simulink model "Assembly_union"  (R2020a)
settings: Solver=VariableStepAuto  StartTime=0.0  StopTime=inf  RelTol=1e-3
model workspace: external: MATLAB File A:\Usuarios\TATTO PC\Desktop\univesidad\Procesamiento video y audio\proyecto 6 intelingencia artificial\Assembly3_DataFile.m (data not in the file)
undefined symbols (not defined in the file or in its folder): smiData, X, Y, Z
libraries: neural x563, sm_lib x153, nesl_utility x4, dspstat3 x3, audiosources x1, simulink x1, dspxfrm3 x1
(part 3 of 36)

== system Assembly_union/Assembly_zona_1/l31_1_RIGID ==
  ReferenceFrame : sm_lib/Frames and Transforms/Reference Frame
  Solid : sm_lib/Body Elements/File Solid  ExtGeomFileName=l31.step  UnitType=FromFile  ExtGeomFileUnits=m  StepReaderType=HEX  ExportConvexHullGeometry=off  InertiaType=Custom  Mass=1  MassUnits=kg  CenterOfMass=smiData.Solid(36).CoM  CenterOfMassUnits=mm  MomentsOfInertia=smiData.Solid(36).MoI  MomentsOfInertiaUnits=kg*mm^2  ProductsOfInertia=smiData.Solid(36).PoI  ProductsOfInertiaUnits=kg*mm^2  BasedOnType=DensityFromFile  Density=1000  DensityUnits=kg/m^3  DoExposeReferenceFrame=on  SerializedFrames=<Frames/>  GraphicType=FromGeometry  MarkerShape=Sphere  MarkerSize=10  GraphicVisPropType=SimpleVisualProperties  GraphicDiffuseColor=[1.0 0.8 0.0]  GraphicSpecularColor=[0.5 0.5 0.5 1.0]  GraphicAmbientColor=[0.15 0.15 0.15 1.0]  GraphicEmissiveColor=[0.0 0.0 0.0 1.0]  GraphicShininess=75  GraphicOpacity=smiData.Solid(36).opacity
  F : PMIOPort  Side=Left
  connections:
  Solid/RConn1 -- ReferenceFrame/RConn1 -- F/RConn1

== system Assembly_union/Assembly_zona_1/l32_1_RIGID ==
  ReferenceFrame : sm_lib/Frames and Transforms/Reference Frame
  Solid : sm_lib/Body Elements/File Solid  ExtGeomFileName=l32.step  UnitType=FromFile  ExtGeomFileUnits=m  StepReaderType=HEX  ExportConvexHullGeometry=off  InertiaType=Custom  Mass=1  MassUnits=kg  CenterOfMass=smiData.Solid(50).CoM  CenterOfMassUnits=mm  MomentsOfInertia=smiData.Solid(50).MoI  MomentsOfInertiaUnits=kg*mm^2  ProductsOfInertia=smiData.Solid(50).PoI  ProductsOfInertiaUnits=kg*mm^2  BasedOnType=DensityFromFile  Density=1000  DensityUnits=kg/m^3  DoExposeReferenceFrame=on  SerializedFrames=<Frames/>  GraphicType=FromGeometry  MarkerShape=Sphere  MarkerSize=10  GraphicVisPropType=SimpleVisualProperties  GraphicDiffuseColor=[1.0 0.8 0.0]  GraphicSpecularColor=[0.5 0.5 0.5 1.0]  GraphicAmbientColor=[0.15 0.15 0.15 1.0]  GraphicEmissiveColor=[0.0 0.0 0.0 1.0]  GraphicShininess=75  GraphicOpacity=smiData.Solid(50).opacity
  F : PMIOPort  Side=Left
  connections:
  Solid/RConn1 -- ReferenceFrame/RConn1 -- F/RConn1

== system Assembly_union/Assembly_zona_1/l41_1_RIGID ==
  ReferenceFrame : sm_lib/Frames and Transforms/Reference Frame
  Solid : sm_lib/Body Elements/File Solid  ExtGeomFileName=l41.step  UnitType=FromFile  ExtGeomFileUnits=m  StepReaderType=HEX  ExportConvexHullGeometry=off  InertiaType=Custom  Mass=1  MassUnits=kg  CenterOfMass=smiData.Solid(39).CoM  CenterOfMassUnits=mm  MomentsOfInertia=smiData.Solid(39).MoI  MomentsOfInertiaUnits=kg*mm^2  ProductsOfInertia=smiData.Solid(39).PoI  ProductsOfInertiaUnits=kg*mm^2  BasedOnType=DensityFromFile  Density=1000  DensityUnits=kg/m^3  DoExposeReferenceFrame=on  SerializedFrames=<Frames/>  GraphicType=FromGeometry  MarkerShape=Sphere  MarkerSize=10  GraphicVisPropType=SimpleVisualProperties  GraphicDiffuseColor=[1.0 0.8 0.0]  GraphicSpecularColor=[0.5 0.5 0.5 1.0]  GraphicAmbientColor=[0.15 0.15 0.15 1.0]  GraphicEmissiveColor=[0.0 0.0 0.0 1.0]  GraphicShininess=75  GraphicOpacity=smiData.Solid(39).opacity
  F : PMIOPort  Side=Left
  connections:
  Solid/RConn1 -- ReferenceFrame/RConn1 -- F/RConn1

== system Assembly_union/Assembly_zona_1/l42_1_RIGID ==
  ReferenceFrame : sm_lib/Frames and Transforms/Reference Frame
  Solid : sm_lib/Body Elements/File Solid  ExtGeomFileName=l42.step  UnitType=FromFile  ExtGeomFileUnits=m  StepReaderType=HEX  ExportConvexHullGeometry=off  InertiaType=Custom  Mass=1  MassUnits=kg  CenterOfMass=smiData.Solid(41).CoM  CenterOfMassUnits=mm  MomentsOfInertia=smiData.Solid(41).MoI  MomentsOfInertiaUnits=kg*mm^2  ProductsOfInertia=smiData.Solid(41).PoI  ProductsOfInertiaUnits=kg*mm^2  BasedOnType=DensityFromFile  Density=1000  DensityUnits=kg/m^3  DoExposeReferenceFrame=on  SerializedFrames=<Frames/>  GraphicType=FromGeometry  MarkerShape=Sphere  MarkerSize=10  GraphicVisPropType=SimpleVisualProperties  GraphicDiffuseColor=[1.0 0.8 0.0]  GraphicSpecularColor=[0.5 0.5 0.5 1.0]  GraphicAmbientColor=[0.15 0.15 0.15 1.0]  GraphicEmissiveColor=[0.0 0.0 0.0 1.0]  GraphicShininess=75  GraphicOpacity=smiData.Solid(41).opacity
  F : PMIOPort  Side=Left
  connections:
  Solid/RConn1 -- ReferenceFrame/RConn1 -- F/RConn1

== system Assembly_union/Assembly_zona_1/lineacentro_1_RIGID ==
  ReferenceFrame : sm_lib/Frames and Transforms/Reference Frame
  Solid : sm_lib/Body Elements/File Solid  ExtGeomFileName=lineacentro.step  UnitType=FromFile  ExtGeomFileUnits=m  StepReaderType=HEX  ExportConvexHullGeometry=off  InertiaType=Custom  Mass=1  MassUnits=kg  CenterOfMass=smiData.Solid(45).CoM  CenterOfMassUnits=mm  MomentsOfInertia=smiData.Solid(45).MoI  MomentsOfInertiaUnits=kg*mm^2  ProductsOfInertia=smiData.Solid(45).PoI  ProductsOfInertiaUnits=kg*mm^2  BasedOnType=DensityFromFile  Density=1000  DensityUnits=kg/m^3  DoExposeReferenceFrame=on  SerializedFrames=<Frames/>  GraphicType=FromGeometry  MarkerShape=Sphere  MarkerSize=10  GraphicVisPropType=SimpleVisualProperties  GraphicDiffuseColor=[1.0 0.8 0.0]  GraphicSpecularColor=[0.5 0.5 0.5 1.0]  GraphicAmbientColor=[0.15 0.15 0.15 1.0]  GraphicEmissiveColor=[0.0 0.0 0.0 1.0]  GraphicShininess=75  GraphicOpacity=smiData.Solid(45).opacity
  F : PMIOPort  Side=Left
  connections:
  Solid/RConn1 -- ReferenceFrame/RConn1 -- F/RConn1

== system Assembly_union/Assembly_zona_1/pasto1_1_RIGID ==
  ReferenceFrame : sm_lib/Frames and Transforms/Reference Frame
  Solid : sm_lib/Body Elements/File Solid  ExtGeomFileName=pasto1.step  UnitType=FromFile  ExtGeomFileUnits=m  StepReaderType=HEX  ExportConvexHullGeometry=off  InertiaType=Custom  Mass=1  MassUnits=kg  CenterOfMass=smiData.Solid(40).CoM  CenterOfMassUnits=mm  MomentsOfInertia=smiData.Solid(40).MoI  MomentsOfInertiaUnits=kg*mm^2  ProductsOfInertia=smiData.Solid(40).PoI  ProductsOfInertiaUnits=kg*mm^2  BasedOnType=DensityFromFile  Density=1000  DensityUnits=kg/m^3  DoExposeReferenceFrame=on  SerializedFrames=<Frames/>  GraphicType=FromGeometry  MarkerShape=Sphere  MarkerSize=10  GraphicVisPropType=SimpleVisualProperties  GraphicDiffuseColor=[0.2 0.6 0.0]  GraphicSpecularColor=[0.5 0.5 0.5 1.0]  GraphicAmbientColor=[0.15 0.15 0.15 1.0]  GraphicEmissiveColor=[0.0 0.0 0.0 1.0]  GraphicShininess=75  GraphicOpacity=smiData.Solid(40).opacity
  F : PMIOPort  Side=Left
  connections:
  Solid/RConn1 -- ReferenceFrame/RConn1 -- F/RConn1

== system Assembly_union/Assembly_zona_1/pasto2_1_RIGID ==
  ReferenceFrame : sm_lib/Frames and Transforms/Reference Frame
  Solid : sm_lib/Body Elements/File Solid  ExtGeomFileName=pasto2.step  UnitType=FromFile  ExtGeomFileUnits=m  StepReaderType=HEX  ExportConvexHullGeometry=off  InertiaType=Custom  Mass=1  MassUnits=kg  CenterOfMass=smiData.Solid(42).CoM  CenterOfMassUnits=mm  MomentsOfInertia=smiData.Solid(42).MoI  MomentsOfInertiaUnits=kg*mm^2  ProductsOfInertia=smiData.Solid(42).PoI  ProductsOfInertiaUnits=kg*mm^2  BasedOnType=DensityFromFile  Density=1000  DensityUnits=kg/m^3  DoExposeReferenceFrame=on  SerializedFrames=<Frames/>  GraphicType=FromGeometry  MarkerShape=Sphere  MarkerSize=10  GraphicVisPropType=SimpleVisualProperties  GraphicDiffuseColor=[0.2 0.6 0.0]  GraphicSpecularColor=[0.5 0.5 0.5 1.0]  GraphicAmbientColor=[0.15 0.15 0.15 1.0]  GraphicEmissiveColor=[0.0 0.0 0.0 1.0]  GraphicShininess=75  GraphicOpacity=smiData.Solid(42).opacity
  F : PMIOPort  Side=Left
  connections:
  Solid/RConn1 -- ReferenceFrame/RConn1 -- F/RConn1

== system Assembly_union/Assembly_zona_1/pasto4_1_RIGID ==
  ReferenceFrame : sm_lib/Frames and Transforms/Reference Frame
  Solid : sm_lib/Body Elements/File Solid  ExtGeomFileName=pasto4.step  UnitType=FromFile  ExtGeomFileUnits=m  StepReaderType=HEX  ExportConvexHullGeometry=off  InertiaType=Custom  Mass=1  MassUnits=kg  CenterOfMass=smiData.Solid(52).CoM  CenterOfMassUnits=mm  MomentsOfInertia=smiData.Solid(52).MoI  MomentsOfInertiaUnits=kg*mm^2  ProductsOfInertia=smiData.Solid(52).PoI  ProductsOfInertiaUnits=kg*mm^2  BasedOnType=DensityFromFile  Density=1000  DensityUnits=kg/m^3  DoExposeReferenceFrame=on  SerializedFrames=<Frames/>  GraphicType=FromGeometry  MarkerShape=Sphere  MarkerSize=10  GraphicVisPropType=SimpleVisualProperties  GraphicDiffuseColor=[0.2 0.6 0.0]  GraphicSpecularColor=[0.5 0.5 0.5 1.0]  GraphicAmbientColor=[0.15 0.15 0.15 1.0]  GraphicEmissiveColor=[0.0 0.0 0.0 1.0]  GraphicShininess=75  GraphicOpacity=smiData.Solid(52).opacity
  F : PMIOPort  Side=Left
  connections:
  Solid/RConn1 -- ReferenceFrame/RConn1 -- F/RConn1

== system Assembly_union/Assembly_zona_1/pasto5_1_RIGID ==
  ReferenceFrame : sm_lib/Frames and Transforms/Reference Frame
  Solid : sm_lib/Body Elements/File Solid  ExtGeomFileName=pasto5.step  UnitType=FromFile  ExtGeomFileUnits=m  StepReaderType=HEX  ExportConvexHullGeometry=off  InertiaType=Custom  Mass=1  MassUnits=kg  CenterOfMass=smiData.Solid(51).CoM  CenterOfMassUnits=mm  MomentsOfInertia=smiData.Solid(51).MoI  MomentsOfInertiaUnits=kg*mm^2  ProductsOfInertia=smiData.Solid(51).PoI  ProductsOfInertiaUnits=kg*mm^2  BasedOnType=DensityFromFile  Density=1000  DensityUnits=kg/m^3  DoExposeReferenceFrame=on  SerializedFrames=<Frames/>  GraphicType=FromGeometry  MarkerShape=Sphere  MarkerSize=10  GraphicVisPropType=SimpleVisualProperties  GraphicDiffuseColor=[0.2 0.6 0.0]  GraphicSpecularColor=[0.5 0.5 0.5 1.0]  GraphicAmbientColor=[0.15 0.15 0.15 1.0]  GraphicEmissiveColor=[0.0 0.0 0.0 1.0]  GraphicShininess=75  GraphicOpacity=smiData.Solid(51).opacity
  F : PMIOPort  Side=Left
  connections:
  Solid/RConn1 -- ReferenceFrame/RConn1 -- F/RConn1

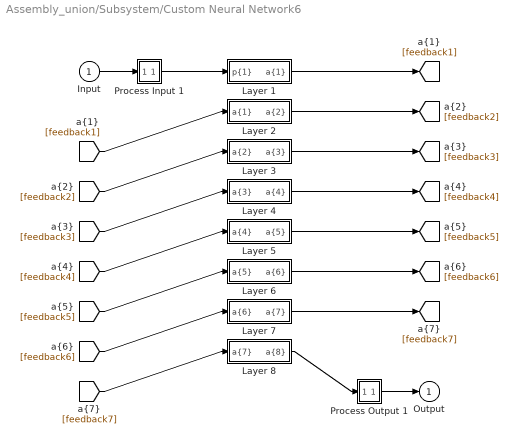
== system Assembly_union/Subsystem/Custom Neural Network6 ==
  Input : Inport  PortDimensions=63
      mask Display: e = 0.06;c1 = [120 230 180]/255;c2 = ([120 230 180]+0)/(256+128);c3 = ([120 230 180]+128)/(256+128);patch([0 1 1 0],[0 0 1 1],c1);patch([0 1 1 1-e 1-e 0+e],[0 0 1 1-e 0+e 0+e],c2);patch([0 0 1 1-e 0+e 0+e],[0 1 1 1-e 1-e 0+e],c3);plot([0 1 1 0 0],[0 0 1 1 0]);
  Layer 1 : Subsystem
      mask Display: e = 0.06;c1 = [120 150 230]/255;c2 = ([120 150 230]+0)/383;c3 = ([120 150 230]+128)/383;patch([0 1 1 0],[0 0 1 1],c1);patch([0 1 1 1-e 1-e 0+e],[0 0 1 1-e 0+e 0+e],c2);patch([0 0 1 1-e 0+e 0+e],[0 1 1 1-e 1-e 0+e],c3);plot([0 1 1 0 0],[0 0 1 1 0]);
  Layer 2 : Subsystem
      mask Display: e = 0.06;c1 = [120 150 230]/255;c2 = ([120 150 230]+0)/383;c3 = ([120 150 230]+128)/383;patch([0 1 1 0],[0 0 1 1],c1);patch([0 1 1 1-e 1-e 0+e],[0 0 1 1-e 0+e 0+e],c2);patch([0 0 1 1-e 0+e 0+e],[0 1 1 1-e 1-e 0+e],c3);plot([0 1 1 0 0],[0 0 1 1 0]);
  Layer 3 : Subsystem
      mask Display: e = 0.06;c1 = [120 150 230]/255;c2 = ([120 150 230]+0)/383;c3 = ([120 150 230]+128)/383;patch([0 1 1 0],[0 0 1 1],c1);patch([0 1 1 1-e 1-e 0+e],[0 0 1 1-e 0+e 0+e],c2);patch([0 0 1 1-e 0+e 0+e],[0 1 1 1-e 1-e 0+e],c3);plot([0 1 1 0 0],[0 0 1 1 0]);
  Layer 4 : Subsystem
      mask Display: e = 0.06;c1 = [120 150 230]/255;c2 = ([120 150 230]+0)/383;c3 = ([120 150 230]+128)/383;patch([0 1 1 0],[0 0 1 1],c1);patch([0 1 1 1-e 1-e 0+e],[0 0 1 1-e 0+e 0+e],c2);patch([0 0 1 1-e 0+e 0+e],[0 1 1 1-e 1-e 0+e],c3);plot([0 1 1 0 0],[0 0 1 1 0]);
  Layer 5 : Subsystem
      mask Display: e = 0.06;c1 = [120 150 230]/255;c2 = ([120 150 230]+0)/383;c3 = ([120 150 230]+128)/383;patch([0 1 1 0],[0 0 1 1],c1);patch([0 1 1 1-e 1-e 0+e],[0 0 1 1-e 0+e 0+e],c2);patch([0 0 1 1-e 0+e 0+e],[0 1 1 1-e 1-e 0+e],c3);plot([0 1 1 0 0],[0 0 1 1 0]);
  Layer 6 : Subsystem
      mask Display: e = 0.06;c1 = [120 150 230]/255;c2 = ([120 150 230]+0)/383;c3 = ([120 150 230]+128)/383;patch([0 1 1 0],[0 0 1 1],c1);patch([0 1 1 1-e 1-e 0+e],[0 0 1 1-e 0+e 0+e],c2);patch([0 0 1 1-e 0+e 0+e],[0 1 1 1-e 1-e 0+e],c3);plot([0 1 1 0 0],[0 0 1 1 0]);
  Layer 7 : Subsystem
      mask Display: e = 0.06;c1 = [120 150 230]/255;c2 = ([120 150 230]+0)/383;c3 = ([120 150 230]+128)/383;patch([0 1 1 0],[0 0 1 1],c1);patch([0 1 1 1-e 1-e 0+e],[0 0 1 1-e 0+e 0+e],c2);patch([0 0 1 1-e 0+e 0+e],[0 1 1 1-e 1-e 0+e],c3);plot([0 1 1 0 0],[0 0 1 1 0]);
  Layer 8 : Subsystem
      mask Display: e = 0.06;c1 = [120 150 230]/255;c2 = ([120 150 230]+0)/383;c3 = ([120 150 230]+128)/383;patch([0 1 1 0],[0 0 1 1],c1);patch([0 1 1 1-e 1-e 0+e],[0 0 1 1-e 0+e 0+e],c2);patch([0 0 1 1-e 0+e 0+e],[0 1 1 1-e 1-e 0+e],c3);plot([0 1 1 0 0],[0 0 1 1 0]);
  Process Input 1 : Subsystem
      mask Display: e = 0.06;c1 = [120 150 230]/255;c2 = ([120 150 230]+0)/383;c3 = ([120 150 230]+128)/383;patch([0 1 1 0],[0 0 1 1],c1);patch([0 1 1 1-e 1-e 0+e],[0 0 1 1-e 0+e 0+e],c2);patch([0 0 1 1-e 0+e 0+e],[0 1 1 1-e 1-e 0+e],c3);plot([0 1 1 0 0],[0 0 1 1 0]);
  Process Output 1 : Subsystem
      mask Display: e = 0.06;c1 = [120 150 230]/255;c2 = ([120 150 230]+0)/383;c3 = ([120 150 230]+128)/383;patch([0 1 1 0],[0 0 1 1],c1);patch([0 1 1 1-e 1-e 0+e],[0 0 1 1-e 0+e 0+e],c2);patch([0 0 1 1-e 0+e 0+e],[0 1 1 1-e 1-e 0+e],c3);plot([0 1 1 0 0],[0 0 1 1 0]);
  Output : Outport  InitialOutput=[0;0;0;0;0;0;0;0;0;0;0;0;0;0;0;0;0;0;0;0;0;0;0;0;0;0;0;0;0;0;0;0;0;0;0;0;0;0;0;0;0;0;0;0;0;0;0;0;0;0;0;0;0;0;0;0;0;0;0;0;0;0;0]
      mask Display: e = 0.06;c1 = [120 230 180]/255;c2 = ([120 230 180]+0)/(256+128);c3 = ([120 230 180]+128)/(256+128);patch([0 1 1 0],[0 0 1 1],c1);patch([0 1 1 1-e 1-e 0+e],[0 0 1 1-e 0+e 0+e],c2);patch([0 0 1 1-e 0+e 0+e],[0 1 1 1-e 1-e 0+e],c3);plot([0 1 1 0 0],[0 0 1 1 0]);
  wires:
  Input/1 -> Process Input 1/1(x)
  Process Output 1/1(y) -> Output/1
  Process Input 1/1(p) -> Layer 1/1("p{1}")
  Layer 1/1("a{1}") -> [feedback1]
  [feedback1] -> Layer 2/1("a{1} ")
  Layer 2/1("a{2}") -> [feedback2]
  [feedback2] -> Layer 3/1("a{2} ")
  Layer 3/1("a{3}") -> [feedback3]
  [feedback3] -> Layer 4/1("a{3} ")
  Layer 4/1("a{4}") -> [feedback4]
  [feedback4] -> Layer 5/1("a{4} ")
  Layer 5/1("a{5}") -> [feedback5]
  [feedback5] -> Layer 6/1("a{5} ")
  Layer 6/1("a{6}") -> [feedback6]
  [feedback6] -> Layer 7/1("a{6} ")
  Layer 7/1("a{7}") -> [feedback7]
  [feedback7] -> Layer 8/1("a{7} ")
  Layer 8/1("a{8}") -> Process Output 1/1(a)

== system Assembly_union/Subsystem/Custom Neural Network6/Layer 1 ==
  "p{1}" : Inport  PortDimensions=63
      mask Display: e = 0.06;c1 = [120 230 180]/255;c2 = ([120 230 180]+0)/(256+128);c3 = ([120 230 180]+128)/(256+128);patch([0 1 1 0],[0 0 1 1],c1);patch([0 1 1 1-e 1-e 0+e],[0 0 1 1-e 0+e 0+e],c2);patch([0 0 1 1-e 0+e 0+e],[0 1 1 1-e 1-e 0+e],c3);plot([0 1 1 0 0],[0 0 1 1 0]);
  Delays 1 : Subsystem
      mask Display: e = 0.06;c1 = [120 150 230]/255;c2 = ([120 150 230]+0)/383;c3 = ([120 150 230]+128)/383;patch([0 1 1 0],[0 0 1 1],c1);patch([0 1 1 1-e 1-e 0+e],[0 0 1 1-e 0+e 0+e],c2);patch([0 0 1 1-e 0+e 0+e],[0 1 1 1-e 1-e 0+e],c3);plot([0 1 1 0 0],[0 0 1 1 0]);disp('0');
  "IW{1,1}" : Subsystem
      mask Display: e = 0.06;c1 = [120 150 230]/255;c2 = ([120 150 230]+0)/383;c3 = ([120 150 230]+128)/383;patch([0 1 1 0],[0 0 1 1],c1);patch([0 1 1 1-e 1-e 0+e],[0 0 1 1-e 0+e 0+e],c2);patch([0 0 1 1-e 0+e 0+e],[0 1 1 1-e 1-e 0+e],c3);plot([0 1 1 0 0],[0 0 1 1 0]);disp('W');
  "b{1}" : Constant  Value=[-1.550357727038423671928057956392876803874969482421875;1.4470399743728241670481793335056863725185394287109375;-1.4617342382418410107192130453768186271190643310546875;1.3544264579599758491212924127466976642608642578125;-1.332780594198820001139438318205066025257110595703125;-1.281869263495257538210125858313404023647308349609375;-1.2429855642347249489176874703844077885150909423828125;1.1965614301382865303224889430566690862178802490234375;1.150447237016904100670444677234627306461334228515625;1.1076856284415625975015018411795608699321746826171875;-1.0671947287690344285948640390415675938129425048828125;-1.0218377385453776273749326719553209841251373291015625;0.9791302377141992696607530888286419212818145751953125;-0.92970916794972235930316628582659177482128143310546875;0.88277326608969708399143883070792071521282196044921875;0.85259394630971219175563646786031313240528106689453125;-0.797070887827824758886663403245620429515838623046875;0.7627876456740059207817239439464174211025238037109375;0.7170558634775912043579637611401267349720001220703125;0.68509918117150625516131867698277346789836883544921875;-0.657791786147828627662192957359366118907928466796875;0.5674359665739194813482981771812774240970611572265625;-0.54259375737416493112874604776152409613132476806640625;-0.51667223145751706159245486560394056141376495361328125;-0.454104607036566798594634519758983515202999114990234375;-0.41485030802403743965811599991866387426853179931640625;-0.35684593574554834827239346850547008216381072998046875;0.32771899110818070166573079404770396649837493896484375;0.25727155434146009582718761521391570568084716796875;-0.2334452069519412920062251259878394193947315216064453125;-0.1877030549718397001157654813141562044620513916015625;0.15072051773341854641330428421497344970703125;-0.10889311824829679686832406559915398247539997100830078125;0.050491628255018468351966731688662548549473285675048828125;0.0192865747800914366649749354110099375247955322265625;-0.022123242606346064931255313013025443069636821746826171875;-0.05263233856318709491528551325245643965899944305419921875;-0.11632565292821432645364865265946718864142894744873046875;0.1708024797534551109112754829766345210373401641845703125;0.1878478259147150775110191034400486387312412261962890625;-0.2442854221391420888043199965977692045271396636962890625;-0.2809311906560338911731378175318241119384765625;-0.322760707928959167389848516904748976230621337890625;-0.369668965987821118712730594779714010655879974365234375;-0.41898239754938793044658496000920422375202178955078125;0.458632299767689488589894608594477176666259765625;0.495758476221943078510179248041822575032711029052734375;-0.51115983647028973013703989636269398033618927001953125;-0.5699831976077576189965157027472741901874542236328125;0.6242764405988110443246341674239374697208404541015625;0.69164310496723213628200710445526055991649627685546875;-0.705583374553743869483923845109529793262481689453125;-0.77264797713766519837719215502147562801837921142578125;-0.793747601233798061315383165492676198482513427734375;0.82215014987183610006837852779426611959934234619140625;0.88353905011437616767722147415042854845523834228515625;-0.9455945735740918234313312495942227542400360107421875;-0.99019652083277076570766439544968307018280029296875;1.0171662055149415238020083052106201648712158203125;1.0700968569369597727103382567293010652065277099609375;-1.1381989868155120149140202556736767292022705078125;-1.15638637640822761198933221749030053615570068359375;-1.2248723353568939931079739835695363581180572509765625;1.2403596519018755817143073727493174374103546142578125;1.2795648758247690768286020102095790207386016845703125;1.321774707896936629225592696457169950008392333984375;-1.3745608698744093967292201341479085385799407958984375;1.4229278619727352417356769365142099559307098388671875;-1.4703002760689154460038707838975824415683746337890625;1.530732570996612640357170675997622311115264892578125]
      mask Display: e = 0.06;c1 = [120 150 230]/255;c2 = ([120 150 230]+0)/383;c3 = ([120 150 230]+128)/383;patch([0 1 1 0],[0 0 1 1],c1);patch([0 1 1 1-e 1-e 0+e],[0 0 1 1-e 0+e 0+e],c2);patch([0 0 1 1-e 0+e 0+e],[0 1 1 1-e 1-e 0+e],c3);plot([0 1 1 0 0],[0 0 1 1 0]);disp('b');
  netsum : Sum  Inputs=2  InputSameDT=on  SaturateOnIntegerOverflow=on  OutDataTypeStr=Inherit: Same as first input
      mask Display: e = 0.06;c1 = [120 150 230]/255;c2 = ([120 150 230]+0)/383;c3 = ([120 150 230]+128)/383;patch([0 1 1 0],[0 0 1 1],c1);patch([0 1 1 1-e 1-e 0+e],[0 0 1 1-e 0+e 0+e],c2);patch([0 0 1 1-e 0+e 0+e],[0 1 1 1-e 1-e 0+e],c3);plot([0 1 1 0 0],[0 0 1 1 0]);disp('+');
  tansig : neural/Transfer Functions/tansig
  "a{1}" : Outport  InitialOutput=[0;0;0;0;0;0;0;0;0;0;0;0;0;0;0;0;0;0;0;0;0;0;0;0;0;0;0;0;0;0;0;0;0;0;0;0;0;0;0;0;0;0;0;0;0;0;0;0;0;0;0;0;0;0;0;0;0;0;0;0;0;0;0;0;0;0;0;0;0;0]
      mask Display: e = 0.06;c1 = [120 230 180]/255;c2 = ([120 230 180]+0)/(256+128);c3 = ([120 230 180]+128)/(256+128);patch([0 1 1 0],[0 0 1 1],c1);patch([0 1 1 1-e 1-e 0+e],[0 0 1 1-e 0+e 0+e],c2);patch([0 0 1 1-e 0+e 0+e],[0 1 1 1-e 1-e 0+e],c3);plot([0 1 1 0 0],[0 0 1 1 0]);
  wires:
  "p{1}"/1 -> Delays 1/1("p{1}")
  Delays 1/1("pd{1,1}") -> "IW{1,1}"/1("pd{1,1}")
  "IW{1,1}"/1("iz{1,1}") -> netsum/1
  "b{1}"/1 -> netsum/2
  netsum/1 -> tansig/1
  tansig/1 -> "a{1}"/1

== system Assembly_union/Subsystem/Custom Neural Network6/Layer 2 ==
  "a{1} " : Inport  PortDimensions=70
      mask Display: e = 0.06;c1 = [120 230 180]/255;c2 = ([120 230 180]+0)/(256+128);c3 = ([120 230 180]+128)/(256+128);patch([0 1 1 0],[0 0 1 1],c1);patch([0 1 1 1-e 1-e 0+e],[0 0 1 1-e 0+e 0+e],c2);patch([0 0 1 1-e 0+e 0+e],[0 1 1 1-e 1-e 0+e],c3);plot([0 1 1 0 0],[0 0 1 1 0]);
  Delays 1 : Subsystem
      mask Display: e = 0.06;c1 = [120 150 230]/255;c2 = ([120 150 230]+0)/383;c3 = ([120 150 230]+128)/383;patch([0 1 1 0],[0 0 1 1],c1);patch([0 1 1 1-e 1-e 0+e],[0 0 1 1-e 0+e 0+e],c2);patch([0 0 1 1-e 0+e 0+e],[0 1 1 1-e 1-e 0+e],c3);plot([0 1 1 0 0],[0 0 1 1 0]);disp('0');
  "LW{2,1}" : Subsystem
      mask Display: e = 0.06;c1 = [120 150 230]/255;c2 = ([120 150 230]+0)/383;c3 = ([120 150 230]+128)/383;patch([0 1 1 0],[0 0 1 1],c1);patch([0 1 1 1-e 1-e 0+e],[0 0 1 1-e 0+e 0+e],c2);patch([0 0 1 1-e 0+e 0+e],[0 1 1 1-e 1-e 0+e],c3);plot([0 1 1 0 0],[0 0 1 1 0]);disp('W');
  "b{2}" : Constant  Value=[1.486726141153912994496977262315340340137481689453125;-1.4442907853435773546380005427636206150054931640625;-1.3994382199420620782603918996755965054035186767578125;1.3639489940170228532423379874671809375286102294921875;-1.313064173078837715280542397522367537021636962890625;-1.253979722265409879611297583323903381824493408203125;1.2320309107327209741100659812218509614467620849609375;-1.1994843709907707651751707089715637266635894775390625;1.1415421256358466717273358881357125937938690185546875;-1.1132711162864368237279677487094886600971221923828125;-1.0368331200875104958214478756417520344257354736328125;1.0218351117924004967107975971885025501251220703125;-0.94548852289680607174915394352865405380725860595703125;-0.939163356491530265657274867407977581024169921875;-0.89687245952084293509898316187900491058826446533203125;-0.84208100302565169759105856428504921495914459228515625;-0.79008406747387860402653814162476919591426849365234375;0.7504057562187711472034834514488466084003448486328125;0.69951147721582784821947598175029270350933074951171875;0.66872624632760935270425761700607836246490478515625;0.61790533552333026801051119036856107413768768310546875;-0.5964692178183546023007011172012425959110260009765625;-0.55270373980923126477904361308901570737361907958984375;-0.494761620773593591149364101511309854686260223388671875;-0.459687958993470979773832141290768049657344818115234375;-0.382591923718393400744020027559599839150905609130859375;0.374736436947102402594822478931746445596218109130859375;0.32834752417064116958300701298867352306842803955078125;-0.259761298706372822930887878101202659308910369873046875;0.243978329773085478304750495226471684873104095458984375;-0.2013183391247168885218599143627216108143329620361328125;-0.135075152550246435634306862993980757892131805419921875;0.09967379369076879991329320773729705251753330230712890625;0.07715536331574927852994250088158878497779369354248046875;0.0254663908700082895764094104151809005998075008392333984375;0.01311071261576543349469670118878639186732470989227294921875;0.08649478978454593069979949859771295450627803802490234375;-0.10679916289935420525836207161773927509784698486328125;0.1416173543784224053698750367402681149542331695556640625;-0.1978407897073064802828668007350643165409564971923828125;0.23368078724311602822893974007456563413143157958984375;0.28895186307564257877089630710543133318424224853515625;-0.325627842263375433251582080629304982721805572509765625;-0.356037176580408232240415600244887173175811767578125;0.423914235533638883435259003817918710410594940185546875;0.449368997809631298689936329537886194884777069091796875;0.50535496942426993971508863978669978678226470947265625;0.55113055039301439563814710709266364574432373046875;0.59100823243280931063026173433172516524791717529296875;-0.6352041961439887085560940249706618487834930419921875;0.66847616649831997914787962145055644214153289794921875;-0.7075611568129236417235006229020655155181884765625;-0.7386605460025419400693635907373391091823577880859375;0.80406440989228122884213689758325926959514617919921875;0.83301432776110073685771340024075470864772796630859375;0.85832211339386343951218805159442126750946044921875;0.9101257219447835833392446147627197206020355224609375;-0.93686181191686301872323383577167987823486328125;-1.01666218669575147970363104832358658313751220703125;-1.057844876234991904340176915866322815418243408203125;-1.1089896128049208101629119482822716236114501953125;1.1414191925987697828759337426163256168365478515625;-1.1843126675446791207235719411983154714107513427734375;1.2263680992950691805987162297242321074008941650390625;1.2703890144356531077818317498895339667797088623046875;-1.3185457817037036232221680620568804442882537841796875;1.3587844545992304734483013817225582897663116455078125;1.4039510047143723969753636993118561804294586181640625;-1.44427349025922868719362668343819677829742431640625;1.472144176816463367885035040671937167644500732421875]
      mask Display: e = 0.06;c1 = [120 150 230]/255;c2 = ([120 150 230]+0)/383;c3 = ([120 150 230]+128)/383;patch([0 1 1 0],[0 0 1 1],c1);patch([0 1 1 1-e 1-e 0+e],[0 0 1 1-e 0+e 0+e],c2);patch([0 0 1 1-e 0+e 0+e],[0 1 1 1-e 1-e 0+e],c3);plot([0 1 1 0 0],[0 0 1 1 0]);disp('b');
  netsum : Sum  Inputs=2  InputSameDT=on  SaturateOnIntegerOverflow=on  OutDataTypeStr=Inherit: Same as first input
      mask Display: e = 0.06;c1 = [120 150 230]/255;c2 = ([120 150 230]+0)/383;c3 = ([120 150 230]+128)/383;patch([0 1 1 0],[0 0 1 1],c1);patch([0 1 1 1-e 1-e 0+e],[0 0 1 1-e 0+e 0+e],c2);patch([0 0 1 1-e 0+e 0+e],[0 1 1 1-e 1-e 0+e],c3);plot([0 1 1 0 0],[0 0 1 1 0]);disp('+');
  tansig : neural/Transfer Functions/tansig
  "a{2}" : Outport  InitialOutput=[0;0;0;0;0;0;0;0;0;0;0;0;0;0;0;0;0;0;0;0;0;0;0;0;0;0;0;0;0;0;0;0;0;0;0;0;0;0;0;0;0;0;0;0;0;0;0;0;0;0;0;0;0;0;0;0;0;0;0;0;0;0;0;0;0;0;0;0;0;0]
      mask Display: e = 0.06;c1 = [120 230 180]/255;c2 = ([120 230 180]+0)/(256+128);c3 = ([120 230 180]+128)/(256+128);patch([0 1 1 0],[0 0 1 1],c1);patch([0 1 1 1-e 1-e 0+e],[0 0 1 1-e 0+e 0+e],c2);patch([0 0 1 1-e 0+e 0+e],[0 1 1 1-e 1-e 0+e],c3);plot([0 1 1 0 0],[0 0 1 1 0]);
  wires:
  "a{1} "/1 -> Delays 1/1("p{2}")
  Delays 1/1("pd{2,1}") -> "LW{2,1}"/1("ad{2,1}")
  "LW{2,1}"/1("lz{2,1}") -> netsum/1
  "b{2}"/1 -> netsum/2
  netsum/1 -> tansig/1
  tansig/1 -> "a{2}"/1

== system Assembly_union/Subsystem/Custom Neural Network6/Layer 3 ==
  "a{2} " : Inport  PortDimensions=70
      mask Display: e = 0.06;c1 = [120 230 180]/255;c2 = ([120 230 180]+0)/(256+128);c3 = ([120 230 180]+128)/(256+128);patch([0 1 1 0],[0 0 1 1],c1);patch([0 1 1 1-e 1-e 0+e],[0 0 1 1-e 0+e 0+e],c2);patch([0 0 1 1-e 0+e 0+e],[0 1 1 1-e 1-e 0+e],c3);plot([0 1 1 0 0],[0 0 1 1 0]);
  Delays 1 : Subsystem
      mask Display: e = 0.06;c1 = [120 150 230]/255;c2 = ([120 150 230]+0)/383;c3 = ([120 150 230]+128)/383;patch([0 1 1 0],[0 0 1 1],c1);patch([0 1 1 1-e 1-e 0+e],[0 0 1 1-e 0+e 0+e],c2);patch([0 0 1 1-e 0+e 0+e],[0 1 1 1-e 1-e 0+e],c3);plot([0 1 1 0 0],[0 0 1 1 0]);disp('0');
  "LW{3,2}" : Subsystem
      mask Display: e = 0.06;c1 = [120 150 230]/255;c2 = ([120 150 230]+0)/383;c3 = ([120 150 230]+128)/383;patch([0 1 1 0],[0 0 1 1],c1);patch([0 1 1 1-e 1-e 0+e],[0 0 1 1-e 0+e 0+e],c2);patch([0 0 1 1-e 0+e 0+e],[0 1 1 1-e 1-e 0+e],c3);plot([0 1 1 0 0],[0 0 1 1 0]);disp('W');
  "b{3}" : Constant  Value=[-1.478712157836084895023986973683349788188934326171875;-1.44204025517263811906332193757407367229461669921875;-1.406160436295465832046147625078447163105010986328125;1.349848375515560139348281154525466263294219970703125;1.3156653068339687617793742901994846761226654052734375;-1.2762747774459175520433973360923118889331817626953125;-1.216296923068817203983371655340306460857391357421875;-1.1936907194513113328326880946406163275241851806640625;1.1221280139287930222025124749052338302135467529296875;-1.0837860130475418518614105778397060930728912353515625;1.0362053873025127703755288166576065123081207275390625;-1.0085725426768890056195004945038817822933197021484375;0.97819503990188894082535853158333338797092437744140625;0.92446207740053953916259388279286213219165802001953125;-0.8904274695234712933000764678581617772579193115234375;-0.84085790275626559608923571431660093367099761962890625;0.78919718103128222441711159262922592461109161376953125;-0.75497647689017532979249835989321582019329071044921875;-0.70744719782572296207234785470063798129558563232421875;-0.67212498236491058367647610793937928974628448486328125;0.62391315929321589095479794195853173732757568359375;-0.58838687733364880561026666327961720526218414306640625;0.557943690780818624119774540304206311702728271484375;0.484293768076833830438232553206034936010837554931640625;-0.466714954829699102401008303786511532962322235107421875;0.408588143869419162523826116739655844867229461669921875;-0.370041780411621779034447854428435675799846649169921875;0.317845037801988639092343191805412061512470245361328125;0.285718702158025250614770129686803556978702545166015625;0.2279027705901833511514809060827246867120265960693359375;0.197681625942910443871625147949089296162128448486328125;0.141639221770150924850639739815960638225078582763671875;0.10991122798684893613341273521655239164829254150390625;-0.08405459902338958955159142760749091394245624542236328125;0.0254161748108656902755964068774119368754327297210693359375;0.0030851085640731580085616148068083930411376059055328369140625;-0.053561414881620007799600813314100378192961215972900390625;-0.1067284117360653705741668773043784312903881072998046875;-0.1420466952227823487220348397386260330677032470703125;-0.178821125963351257315281372939352877438068389892578125;-0.245904734168106264835529373158351518213748931884765625;0.27256549324913847964779733956675045192241668701171875;0.346085716802969900474096220932551659643650054931640625;0.36829035823397660021072397285024635493755340576171875;0.42602159858964927519053844662266783416271209716796875;-0.4433163274960831845561415320844389498233795166015625;-0.487373773709561197708950430751428939402103424072265625;-0.52597012896472083998133939530816860496997833251953125;0.5918245858972175366119472528225742280483245849609375;0.611382544474934785938557979534380137920379638671875;-0.6259379549411037135797641894896514713764190673828125;0.725374415083548829130677404464222490787506103515625;0.75450668920123253879950198097503744065761566162109375;0.79674844577210013341073135961778461933135986328125;-0.84047164760560078011764062466681934893131256103515625;0.88702752590263889143074038656777702271938323974609375;0.92346307374260250266928551354794763028621673583984375;-0.9718546289492600021020507483626715838909149169921875;1.0084743920896108715368200137163512408733367919921875;1.0673275480286650296335437815287150442600250244140625;-1.0968119710053993998144505894742906093597412109375;-1.142154966693210038641836945316754281520843505859375;1.188220600153555128741800217540003359317779541015625;-1.238418755972392926167913174140267074108123779296875;-1.2811983092021359542656000485294498503208160400390625;1.2971547567381327414892666638479568064212799072265625;-1.359799860984459929369450037484057247638702392578125;-1.40312044074937869453378880280070006847381591796875;1.4401144135696120063272473998949863016605377197265625;1.501471035054013913878634411958046257495880126953125]
      mask Display: e = 0.06;c1 = [120 150 230]/255;c2 = ([120 150 230]+0)/383;c3 = ([120 150 230]+128)/383;patch([0 1 1 0],[0 0 1 1],c1);patch([0 1 1 1-e 1-e 0+e],[0 0 1 1-e 0+e 0+e],c2);patch([0 0 1 1-e 0+e 0+e],[0 1 1 1-e 1-e 0+e],c3);plot([0 1 1 0 0],[0 0 1 1 0]);disp('b');
  netsum : Sum  Inputs=2  InputSameDT=on  SaturateOnIntegerOverflow=on  OutDataTypeStr=Inherit: Same as first input
      mask Display: e = 0.06;c1 = [120 150 230]/255;c2 = ([120 150 230]+0)/383;c3 = ([120 150 230]+128)/383;patch([0 1 1 0],[0 0 1 1],c1);patch([0 1 1 1-e 1-e 0+e],[0 0 1 1-e 0+e 0+e],c2);patch([0 0 1 1-e 0+e 0+e],[0 1 1 1-e 1-e 0+e],c3);plot([0 1 1 0 0],[0 0 1 1 0]);disp('+');
  tansig : neural/Transfer Functions/tansig
  "a{3}" : Outport  InitialOutput=[0;0;0;0;0;0;0;0;0;0;0;0;0;0;0;0;0;0;0;0;0;0;0;0;0;0;0;0;0;0;0;0;0;0;0;0;0;0;0;0;0;0;0;0;0;0;0;0;0;0;0;0;0;0;0;0;0;0;0;0;0;0;0;0;0;0;0;0;0;0]
      mask Display: e = 0.06;c1 = [120 230 180]/255;c2 = ([120 230 180]+0)/(256+128);c3 = ([120 230 180]+128)/(256+128);patch([0 1 1 0],[0 0 1 1],c1);patch([0 1 1 1-e 1-e 0+e],[0 0 1 1-e 0+e 0+e],c2);patch([0 0 1 1-e 0+e 0+e],[0 1 1 1-e 1-e 0+e],c3);plot([0 1 1 0 0],[0 0 1 1 0]);
  wires:
  "a{2} "/1 -> Delays 1/1("p{3}")
  Delays 1/1("pd{3,2}") -> "LW{3,2}"/1("ad{3,2}")
  "LW{3,2}"/1("lz{3,2}") -> netsum/1
  "b{3}"/1 -> netsum/2
  netsum/1 -> tansig/1
  tansig/1 -> "a{3}"/1

== system Assembly_union/Subsystem/Custom Neural Network6/Layer 4 ==
  "a{3} " : Inport  PortDimensions=70
      mask Display: e = 0.06;c1 = [120 230 180]/255;c2 = ([120 230 180]+0)/(256+128);c3 = ([120 230 180]+128)/(256+128);patch([0 1 1 0],[0 0 1 1],c1);patch([0 1 1 1-e 1-e 0+e],[0 0 1 1-e 0+e 0+e],c2);patch([0 0 1 1-e 0+e 0+e],[0 1 1 1-e 1-e 0+e],c3);plot([0 1 1 0 0],[0 0 1 1 0]);
  Delays 1 : Subsystem
      mask Display: e = 0.06;c1 = [120 150 230]/255;c2 = ([120 150 230]+0)/383;c3 = ([120 150 230]+128)/383;patch([0 1 1 0],[0 0 1 1],c1);patch([0 1 1 1-e 1-e 0+e],[0 0 1 1-e 0+e 0+e],c2);patch([0 0 1 1-e 0+e 0+e],[0 1 1 1-e 1-e 0+e],c3);plot([0 1 1 0 0],[0 0 1 1 0]);disp('0');
  "LW{4,3}" : Subsystem
      mask Display: e = 0.06;c1 = [120 150 230]/255;c2 = ([120 150 230]+0)/383;c3 = ([120 150 230]+128)/383;patch([0 1 1 0],[0 0 1 1],c1);patch([0 1 1 1-e 1-e 0+e],[0 0 1 1-e 0+e 0+e],c2);patch([0 0 1 1-e 0+e 0+e],[0 1 1 1-e 1-e 0+e],c3);plot([0 1 1 0 0],[0 0 1 1 0]);disp('W');
  "b{4}" : Constant  Value=[1.5076205391287189616633668265421874821186065673828125;-1.4454400764673935864124132422148250043392181396484375;-1.397161785664160493780627803062088787555694580078125;-1.3583220349444637964353432835196144878864288330078125;-1.3171629955426222835512817255221307277679443359375;-1.2654189831773283714255740051157772541046142578125;-1.225895245279738698940263930126093327999114990234375;-1.16834039096092556775374760036356747150421142578125;1.1468101635519019065867496465216390788555145263671875;1.09745774049859701193554428755305707454681396484375;1.0439516658008993754691573485615663230419158935546875;1.0185865979571440131934423334314487874507904052734375;-0.95641176497005264689477144202101044356822967529296875;0.91126947294328719539890926171210594475269317626953125;-0.886998331904802927994069250416941940784454345703125;-0.8234638924262582815316591222654096782207489013671875;-0.783363172959019582464179620728828012943267822265625;0.7483182450542980035379514447413384914398193359375;0.71774674395461068865387233017827384173870086669921875;0.66519349088265877778525236863060854375362396240234375;-0.62450948057194699547522986904368735849857330322265625;-0.56763313346006760706785598813439719378948211669921875;0.5194820002575102346753510573762468993663787841796875;-0.47033850536826482535701643428183160722255706787109375;-0.465320416039982698297450269819819368422031402587890625;-0.40050450986524654961584701595711521804332733154296875;0.366276252772025745496620174890267662703990936279296875;0.332853642976636165951020984721253626048564910888671875;0.29616859492819280763598044359241612255573272705078125;-0.244780544104318986686763537363731302320957183837890625;0.196628780808129732804445666261017322540283203125;-0.160227637155226310117228649687604047358036041259765625;-0.09925608451466851056554929755293414928019046783447265625;0.061610634172378477002585128730061114765703678131103515625;-0.0244463143815594301233584673127552377991378307342529296875;0.02553180005264481244875440779651398770511150360107421875;-0.0609366549343008656602904693500022403895854949951171875;0.11219979101187678438567019156835158355534076690673828125;0.1428638606575833580603074324244516901671886444091796875;0.1876276339611566701393030598410405218601226806640625;-0.252625530374786466669689843911328352987766265869140625;0.2767030950303703829007417880347929894924163818359375;0.339408720682780218336205280138528905808925628662109375;0.371622626067612926714645027459482662379741668701171875;-0.416631015628964818109380985333700664341449737548828125;0.456339399459154415605866006444557569921016693115234375;-0.478570635137376576562218133403803221881389617919921875;-0.539857403775162225656458758749067783355712890625;-0.58933904148836846470516093177138827741146087646484375;0.62058785035510666272529078923980705440044403076171875;-0.66293083572840505457435256175813265144824981689453125;0.7031424374129058296745142797590233385562896728515625;0.75467569143736057402094274948467500507831573486328125;-0.80091318161830304944714953307993710041046142578125;-0.8425541670021250428845860369619913399219512939453125;0.896203394914901974033227816107682883739471435546875;-0.93518123141223241656661002707551233470439910888671875;-0.97110822667775431593639723359956406056880950927734375;0.999815924799395627786680051940493285655975341796875;-1.057337551632094641007597601856105029582977294921875;-1.084754176438625261624792983639054000377655029296875;-1.1475994906122106709034369487199001014232635498046875;-1.1857505015850293705881313144345767796039581298828125;1.242192319077707995944592767045833170413970947265625;1.28533576171691610312564080231823027133941650390625;-1.315637352118816494339625933207571506500244140625;1.3621094318186919291946423982153646647930145263671875;-1.39768257197458733998018942656926810741424560546875;-1.44414663216938077283657548832707107067108154296875;-1.4781683970480152812143614937667734920978546142578125]
      mask Display: e = 0.06;c1 = [120 150 230]/255;c2 = ([120 150 230]+0)/383;c3 = ([120 150 230]+128)/383;patch([0 1 1 0],[0 0 1 1],c1);patch([0 1 1 1-e 1-e 0+e],[0 0 1 1-e 0+e 0+e],c2);patch([0 0 1 1-e 0+e 0+e],[0 1 1 1-e 1-e 0+e],c3);plot([0 1 1 0 0],[0 0 1 1 0]);disp('b');
  netsum : Sum  Inputs=2  InputSameDT=on  SaturateOnIntegerOverflow=on  OutDataTypeStr=Inherit: Same as first input
      mask Display: e = 0.06;c1 = [120 150 230]/255;c2 = ([120 150 230]+0)/383;c3 = ([120 150 230]+128)/383;patch([0 1 1 0],[0 0 1 1],c1);patch([0 1 1 1-e 1-e 0+e],[0 0 1 1-e 0+e 0+e],c2);patch([0 0 1 1-e 0+e 0+e],[0 1 1 1-e 1-e 0+e],c3);plot([0 1 1 0 0],[0 0 1 1 0]);disp('+');
  tansig : neural/Transfer Functions/tansig
  "a{4}" : Outport  InitialOutput=[0;0;0;0;0;0;0;0;0;0;0;0;0;0;0;0;0;0;0;0;0;0;0;0;0;0;0;0;0;0;0;0;0;0;0;0;0;0;0;0;0;0;0;0;0;0;0;0;0;0;0;0;0;0;0;0;0;0;0;0;0;0;0;0;0;0;0;0;0;0]
      mask Display: e = 0.06;c1 = [120 230 180]/255;c2 = ([120 230 180]+0)/(256+128);c3 = ([120 230 180]+128)/(256+128);patch([0 1 1 0],[0 0 1 1],c1);patch([0 1 1 1-e 1-e 0+e],[0 0 1 1-e 0+e 0+e],c2);patch([0 0 1 1-e 0+e 0+e],[0 1 1 1-e 1-e 0+e],c3);plot([0 1 1 0 0],[0 0 1 1 0]);
  wires:
  "a{3} "/1 -> Delays 1/1("p{4}")
  Delays 1/1("pd{4,3}") -> "LW{4,3}"/1("ad{4,3}")
  "LW{4,3}"/1("lz{4,3}") -> netsum/1
  "b{4}"/1 -> netsum/2
  netsum/1 -> tansig/1
  tansig/1 -> "a{4}"/1

== system Assembly_union/Subsystem/Custom Neural Network6/Layer 5 ==
  "a{4} " : Inport  PortDimensions=70
      mask Display: e = 0.06;c1 = [120 230 180]/255;c2 = ([120 230 180]+0)/(256+128);c3 = ([120 230 180]+128)/(256+128);patch([0 1 1 0],[0 0 1 1],c1);patch([0 1 1 1-e 1-e 0+e],[0 0 1 1-e 0+e 0+e],c2);patch([0 0 1 1-e 0+e 0+e],[0 1 1 1-e 1-e 0+e],c3);plot([0 1 1 0 0],[0 0 1 1 0]);
  Delays 1 : Subsystem
      mask Display: e = 0.06;c1 = [120 150 230]/255;c2 = ([120 150 230]+0)/383;c3 = ([120 150 230]+128)/383;patch([0 1 1 0],[0 0 1 1],c1);patch([0 1 1 1-e 1-e 0+e],[0 0 1 1-e 0+e 0+e],c2);patch([0 0 1 1-e 0+e 0+e],[0 1 1 1-e 1-e 0+e],c3);plot([0 1 1 0 0],[0 0 1 1 0]);disp('0');
  "LW{5,4}" : Subsystem
      mask Display: e = 0.06;c1 = [120 150 230]/255;c2 = ([120 150 230]+0)/383;c3 = ([120 150 230]+128)/383;patch([0 1 1 0],[0 0 1 1],c1);patch([0 1 1 1-e 1-e 0+e],[0 0 1 1-e 0+e 0+e],c2);patch([0 0 1 1-e 0+e 0+e],[0 1 1 1-e 1-e 0+e],c3);plot([0 1 1 0 0],[0 0 1 1 0]);disp('W');
  "b{5}" : Constant  Value=[1.4913534708448501486799386839265935122966766357421875;-1.4422974195684796772098934525274671614170074462890625;1.4017552719206129996365461920504458248615264892578125;-1.3457837262271115097433948903926648199558258056640625;-1.3178190209418598755064522265456616878509521484375;1.2677171267943923016474627729621715843677520751953125;1.2073010126882717241159070908906869590282440185546875;-1.1752189556032159867271502662333659827709197998046875;1.1450562194434088514327640950796194374561309814453125;1.1112574248288555889274675791966728866100311279296875;-1.057244907623533070051280446932651102542877197265625;1.046866471741549897700451765558682382106781005859375;-0.970099432584443643889926534029655158519744873046875;0.9233235668642552074203422307618893682956695556640625;-0.88387662237986341917661547995521686971187591552734375;-0.8566071450385168706276317607262171804904937744140625;-0.8012393797821377727785829847562126815319061279296875;-0.757196921632417030423312098719179630279541015625;0.71379591916863904810242047460633330047130584716796875;-0.692684139755799233029165407060645520687103271484375;0.6288687242091508533547994375112466514110565185546875;0.572504236613397221589139007846824824810028076171875;0.550432727718561221053050758200697600841522216796875;0.487460734204362144961208969107246957719326019287109375;-0.4361689822178098641103360932902432978153228759765625;0.417935347458838146739168450949364341795444488525390625;0.373930282203827790699079969272133894264698028564453125;-0.3160875626168007102023693732917308807373046875;-0.271998639184047930061893794118077494204044342041015625;-0.240315501627343497403899164055474102497100830078125;-0.2114422678490905649351105921596172265708446502685546875;-0.1494494749627695295846052658816915936768054962158203125;0.10931624238168570484308617096758098341524600982666015625;0.0629929819834859905380852751477505080401897430419921875;0.0254937841438631802859493546975500066764652729034423828125;-0.0428762284540773197516472237111884169280529022216796875;-0.0547400683400570964298736953423940576612949371337890625;0.10980104994544069574313738257842487655580043792724609375;-0.1629681992929138678594114253428415395319461822509765625;0.18650263243445486249783016319270245730876922607421875;-0.233303221912639024981928059787605889141559600830078125;-0.248728517698107609579238896913011558353900909423828125;-0.326036171763393556322085942156263627111911773681640625;0.347698569176673633052132572629489004611968994140625;-0.41890982146428445975772092424449510872364044189453125;-0.4391639079309761495295560962404124438762664794921875;0.52137939546281042435538211066159419715404510498046875;-0.5524655845069565973659564406261779367923736572265625;-0.595671537104291104469666606746613979339599609375;-0.62668840928778468679638535832054913043975830078125;0.6627662365752626794090929251979105174541473388671875;0.678386584408048776140276459045708179473876953125;-0.75854456412207671434089206741191446781158447265625;0.8290160598146310011458126609795726835727691650390625;0.8532481724066787176496973188477568328380584716796875;0.89473526352379828541216966186766512691974639892578125;-0.93012686074836758987061102743609808385372161865234375;0.98087023998005407054989746029605157673358917236328125;1.028051381649948137209094056743197143077850341796875;1.0601867187419065086118052931851707398891448974609375;1.087843289237398369806442133267410099506378173828125;1.13410985610787218291761746513657271862030029296875;1.186780705444840489093394353403709828853607177734375;1.231636719895401466118300959351472556591033935546875;-1.2782462517565009729736402732669375836849212646484375;1.3136589767421129604230145559995435178279876708984375;1.3509638989650694096411598366103135049343109130859375;-1.3989531576658780220867583921062760055065155029296875;-1.4319956800214066472420881837024353444576263427734375;1.487889377586765871086527113220654428005218505859375]
      mask Display: e = 0.06;c1 = [120 150 230]/255;c2 = ([120 150 230]+0)/383;c3 = ([120 150 230]+128)/383;patch([0 1 1 0],[0 0 1 1],c1);patch([0 1 1 1-e 1-e 0+e],[0 0 1 1-e 0+e 0+e],c2);patch([0 0 1 1-e 0+e 0+e],[0 1 1 1-e 1-e 0+e],c3);plot([0 1 1 0 0],[0 0 1 1 0]);disp('b');
  netsum : Sum  Inputs=2  InputSameDT=on  SaturateOnIntegerOverflow=on  OutDataTypeStr=Inherit: Same as first input
      mask Display: e = 0.06;c1 = [120 150 230]/255;c2 = ([120 150 230]+0)/383;c3 = ([120 150 230]+128)/383;patch([0 1 1 0],[0 0 1 1],c1);patch([0 1 1 1-e 1-e 0+e],[0 0 1 1-e 0+e 0+e],c2);patch([0 0 1 1-e 0+e 0+e],[0 1 1 1-e 1-e 0+e],c3);plot([0 1 1 0 0],[0 0 1 1 0]);disp('+');
  tansig : neural/Transfer Functions/tansig
  "a{5}" : Outport  InitialOutput=[0;0;0;0;0;0;0;0;0;0;0;0;0;0;0;0;0;0;0;0;0;0;0;0;0;0;0;0;0;0;0;0;0;0;0;0;0;0;0;0;0;0;0;0;0;0;0;0;0;0;0;0;0;0;0;0;0;0;0;0;0;0;0;0;0;0;0;0;0;0]
      mask Display: e = 0.06;c1 = [120 230 180]/255;c2 = ([120 230 180]+0)/(256+128);c3 = ([120 230 180]+128)/(256+128);patch([0 1 1 0],[0 0 1 1],c1);patch([0 1 1 1-e 1-e 0+e],[0 0 1 1-e 0+e 0+e],c2);patch([0 0 1 1-e 0+e 0+e],[0 1 1 1-e 1-e 0+e],c3);plot([0 1 1 0 0],[0 0 1 1 0]);
  wires:
  "a{4} "/1 -> Delays 1/1("p{5}")
  Delays 1/1("pd{5,4}") -> "LW{5,4}"/1("ad{5,4}")
  "LW{5,4}"/1("lz{5,4}") -> netsum/1
  "b{5}"/1 -> netsum/2
  netsum/1 -> tansig/1
  tansig/1 -> "a{5}"/1
